simulink model "input_shaping"  (R2023b)
settings: Solver=VariableStepAuto  StartTime=0.0  StopTime=50  RelTol=1e-3
libraries: SignalEditorBlockLib x3
settings Model: Creator=David  LastModifiedBy=David
settings RTWCC: GPUComputeCapability=5.0
settings ConfigComp: CovBoundaryAbsTol=1.0e-5

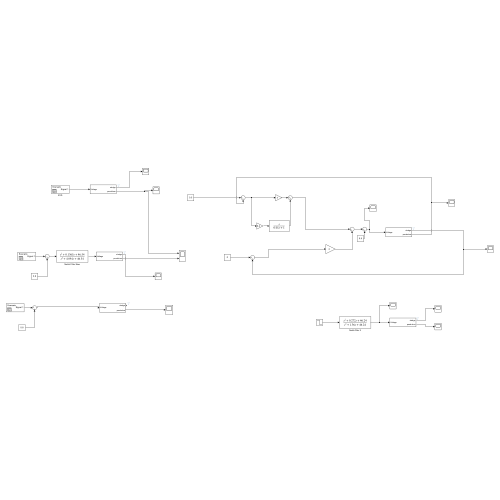
[thumbnail: Simulink's stored preview of the top-level diagram]
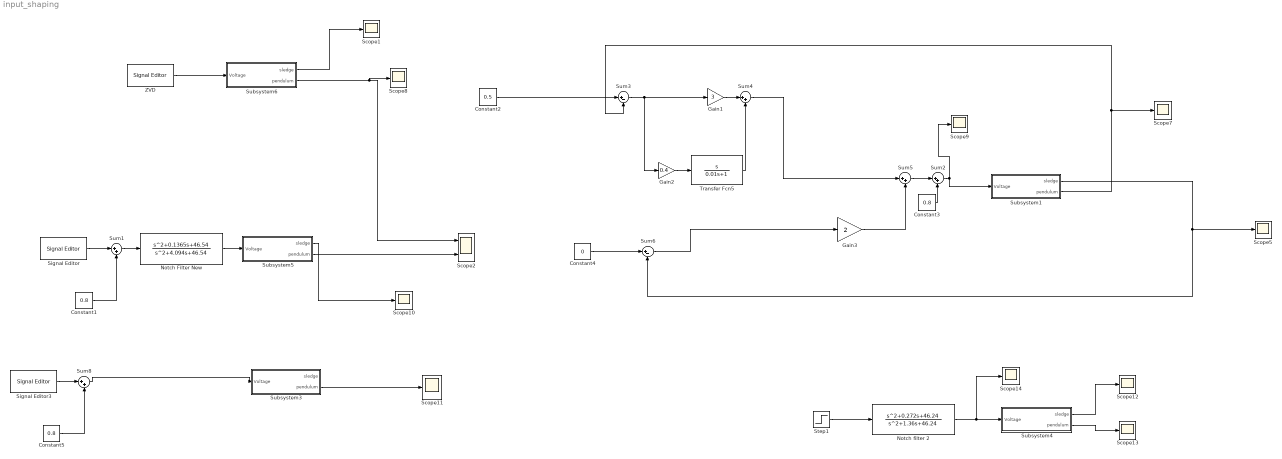
== system input_shaping ==
  Constant1 : Constant  Value=0.8
  Constant2 : Constant  Value=0.5
  Constant3 : Constant  Value=0.8
  Constant4 : Constant  Value=0
  Constant5 : Constant  Value=0.8
  Gain1 : Gain  Gain=3
  Gain2 : Gain  Gain=0.4
  Gain3 : Gain  Gain=2
  Notch Filter New : TransferFcn  Numerator=[1 0.1365 46.54]  Denominator=[1 4.094 46.54]
  Notch filter 2 : TransferFcn  Numerator=[1,0.272,46.24]  Denominator=[1,1.36,46.24]
  Scope{1,5,7..14} (10 alike) : Scope
  Scope2 : Scope  NumInputPorts=2
  Signal Editor : SignalEditorBlockLib/Signal Editor  FileName=ZV.mat  ActiveScenario=Scenario  ActiveSignal=Signal 1  IsBus=off  OutputBusObjectStr=Bus: BusObject  SampleTime=0  ZeroCross=off  OutputAfterFinalValue=Setting to zero  Unit=inherit  PreserveSignalName=on  ApplySigPropsToAllScenarios=on  ApplySigPropsToAllSignals=off
  Signal Editor3 : SignalEditorBlockLib/Signal Editor  FileName=signal_input2.mat  ActiveScenario=Scenario  ActiveSignal=Signal 1  IsBus=off  OutputBusObjectStr=Bus: BusObject  SampleTime=0  ZeroCross=off  OutputAfterFinalValue=Setting to zero  Unit=inherit  PreserveSignalName=on  ApplySigPropsToAllScenarios=on  ApplySigPropsToAllSignals=off
  Step1 : Step  Time=1.5  Before=9  After=0  SampleTime=0
  Subsystem1 : Subsystem
  Subsystem3 : Subsystem
  Subsystem4 : Subsystem
  Subsystem5 : Subsystem
  Subsystem6 : Subsystem
  Sum{1..2,4..5,8} (5 alike) : Sum  Inputs=|++
  Sum3 : Sum  Inputs=|+-
  Sum6 : Sum  Inputs=|+-
  Transfer Fcn5 : TransferFcn  Numerator=[1 0]  Denominator=[0.01 1]
  ZVD : SignalEditorBlockLib/Signal Editor  FileName=signal_input2.mat  ActiveScenario=Scenario  ActiveSignal=Signal 1  IsBus=off  OutputBusObjectStr=Bus: BusObject  SampleTime=0  ZeroCross=off  OutputAfterFinalValue=Setting to zero  Unit=inherit  PreserveSignalName=on  ApplySigPropsToAllScenarios=on  ApplySigPropsToAllSignals=off
  wires:
  Subsystem6/2(pendulum) -> Scope2/1, Scope8/1
  ZVD/1 -> Subsystem6/1(Voltage)
  Constant1/1 -> Sum1/2
  Signal Editor/1 -> Sum1/1
  Sum1/1 -> Notch Filter New/1
  Subsystem5/2(pendulum) -> Scope2/2
  Gain1/1 -> Sum4/1
  Subsystem1/1(sledge) -> Scope5/1, Sum6/2
  Constant2/1 -> Sum3/1
  Subsystem1/2(pendulum) -> Scope7/1, Sum3/2
  Constant3/1 -> Sum2/2
  Subsystem5/1(sledge) -> Scope10/1
  Sum5/1 -> Sum2/1
  Gain3/1 -> Sum5/2
  Constant4/1 -> Sum6/1
  Sum6/1 -> Gain3/1
  Sum3/1 -> Gain2/1, Gain1/1
  Gain2/1 -> Transfer Fcn5/1
  Transfer Fcn5/1 -> Sum4/2
  Signal Editor3/1 -> Sum8/1
  Constant5/1 -> Sum8/2
  Sum8/1 -> Subsystem3/1(Voltage)
  Subsystem3/2(pendulum) -> Scope11/1
  Sum4/1 -> Sum5/1
  Sum2/1 -> Scope9/1, Subsystem1/1(Voltage)
  Step1/1 -> Notch filter 2/1
  Subsystem4/1(sledge) -> Scope12/1
  Subsystem4/2(pendulum) -> Scope13/1
  Notch filter 2/1 -> Scope14/1, Subsystem4/1(Voltage)
  Subsystem6/1(sledge) -> Scope1/1
  Notch Filter New/1 -> Subsystem5/1(Voltage)

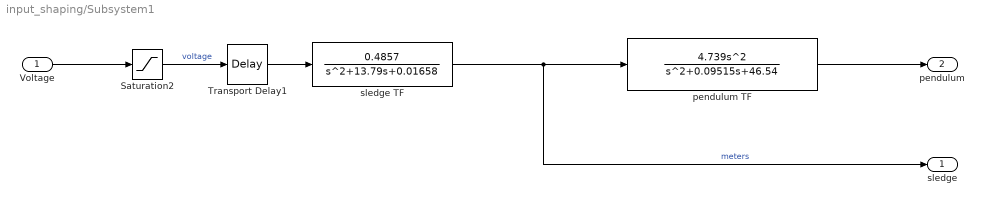
== system input_shaping/Subsystem1 ==
  Voltage : Inport
  Saturation2 : Saturate  UpperLimit=12  LowerLimit=-12
  Transport Delay1 : TransportDelay  DelayTime=0.02
  pendulum TF : TransferFcn  Numerator=[4.739 0 0]  Denominator=[1 0.09515 46.54]
  sledge TF : TransferFcn  Numerator=[0.4857]  Denominator=[1 13.79 0.01658]
  sledge : Outport
  pendulum : Outport  Port=2
  wires:
  Saturation2/1 -> Transport Delay1/1  "voltage"
  sledge TF/1 -> pendulum TF/1, sledge/1  "meters"
  Voltage/1 -> Saturation2/1
  pendulum TF/1 -> pendulum/1
  Transport Delay1/1 -> sledge TF/1

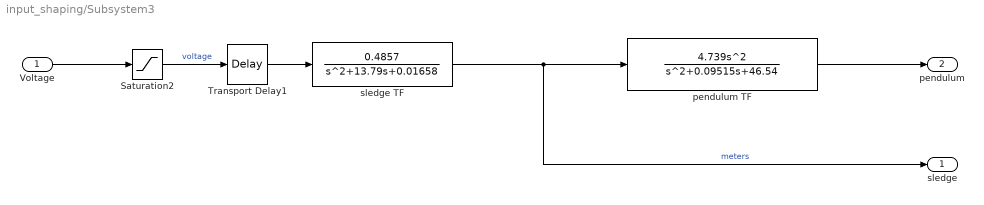
== system input_shaping/Subsystem3 ==
  Voltage : Inport
  Saturation2 : Saturate  UpperLimit=12  LowerLimit=-12
  Transport Delay1 : TransportDelay  DelayTime=0.02
  pendulum TF : TransferFcn  Numerator=[4.739 0 0]  Denominator=[1 0.09515 46.54]
  sledge TF : TransferFcn  Numerator=[0.4857]  Denominator=[1 13.79 0.01658]
  sledge : Outport
  pendulum : Outport  Port=2
  wires:
  Saturation2/1 -> Transport Delay1/1  "voltage"
  sledge TF/1 -> pendulum TF/1, sledge/1  "meters"
  Voltage/1 -> Saturation2/1
  pendulum TF/1 -> pendulum/1
  Transport Delay1/1 -> sledge TF/1

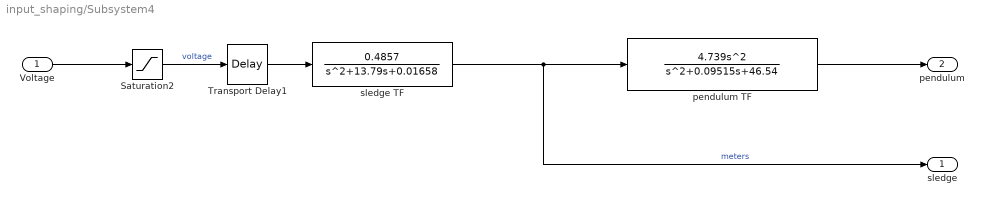
== system input_shaping/Subsystem4 ==
  Voltage : Inport
  Saturation2 : Saturate  UpperLimit=12  LowerLimit=-12
  Transport Delay1 : TransportDelay  DelayTime=0.02
  pendulum TF : TransferFcn  Numerator=[4.739 0 0]  Denominator=[1 0.09515 46.54]
  sledge TF : TransferFcn  Numerator=[0.4857]  Denominator=[1 13.79 0.01658]
  sledge : Outport
  pendulum : Outport  Port=2
  wires:
  Transport Delay1/1 -> sledge TF/1
  pendulum TF/1 -> pendulum/1
  Voltage/1 -> Saturation2/1
  sledge TF/1 -> sledge/1, pendulum TF/1  "meters"
  Saturation2/1 -> Transport Delay1/1  "voltage"

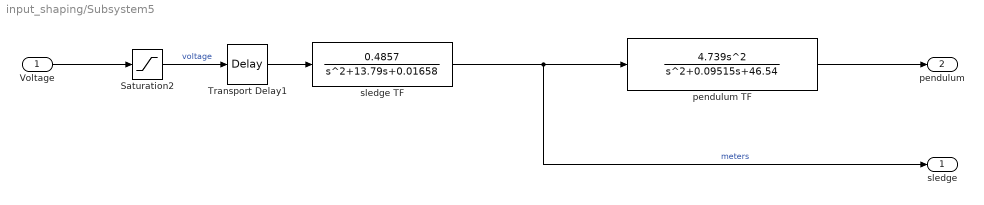
== system input_shaping/Subsystem5 ==
  Voltage : Inport
  Saturation2 : Saturate  UpperLimit=12  LowerLimit=-12
  Transport Delay1 : TransportDelay  DelayTime=0.02
  pendulum TF : TransferFcn  Numerator=[4.739 0 0]  Denominator=[1 0.09515 46.54]
  sledge TF : TransferFcn  Numerator=[0.4857]  Denominator=[1 13.79 0.01658]
  sledge : Outport
  pendulum : Outport  Port=2
  wires:
  Transport Delay1/1 -> sledge TF/1
  pendulum TF/1 -> pendulum/1
  Voltage/1 -> Saturation2/1
  sledge TF/1 -> sledge/1, pendulum TF/1  "meters"
  Saturation2/1 -> Transport Delay1/1  "voltage"

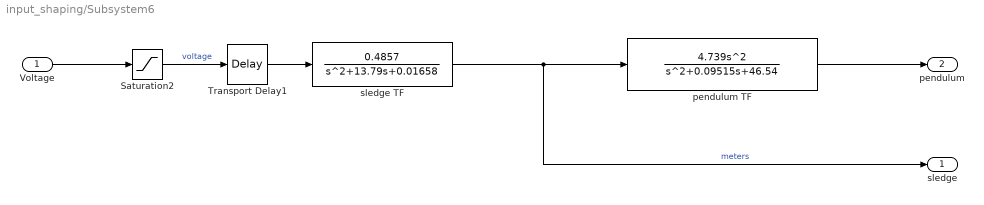
== system input_shaping/Subsystem6 ==
  Voltage : Inport
  Saturation2 : Saturate  UpperLimit=12  LowerLimit=-12
  Transport Delay1 : TransportDelay  DelayTime=0.02
  pendulum TF : TransferFcn  Numerator=[4.739 0 0]  Denominator=[1 0.09515 46.54]
  sledge TF : TransferFcn  Numerator=[0.4857]  Denominator=[1 13.79 0.01658]
  sledge : Outport
  pendulum : Outport  Port=2
  wires:
  Saturation2/1 -> Transport Delay1/1  "voltage"
  sledge TF/1 -> pendulum TF/1, sledge/1  "meters"
  Voltage/1 -> Saturation2/1
  pendulum TF/1 -> pendulum/1
  Transport Delay1/1 -> sledge TF/1
